simulink model "BCM_MBD_External_Lighting"  (R2020b)
settings: Solver=VariableStepAuto  StartTime=0.0  StopTime=50  RelTol=1e-3
undefined symbols (not defined in the file): sigbuilder_block
settings Model: Creator=99003151  LastModifiedBy=99003151

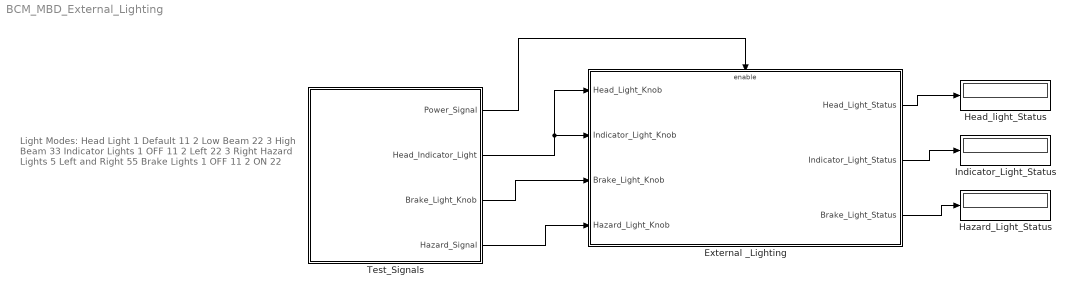
== system BCM_MBD_External_Lighting ==
  note: Light Modes:
      |
      | Head Light
      | 1
      | Default
      | 11
      |
      | 2
      | Low Beam
      | 22
      |
      | 3
      | High Beam
      | 33
      |
      | Indicator Lights
      | 1
      | OFF
      | 11
      |
      | 2
      | Left
      | 22
      |
      | 3
      | Right
      |
      | Hazard Lights
      | 5
      | Left and Right
      | 55
      |
      | Brake Lights
      | 1
      | OFF
      | 11
      |
      | 2
      | ON
      | 22
  External _Lighting : Subsystem  TreatAsAtomicUnit=on
  Hazard_Light_Status : Display
  Head_light_Status : Display
  Indicator_Light_Status : Display
  Test_Signals : Subsystem  Tag=STV Subsys  LoadFcn=sigbuilder_block('load');  StartFcn=sigbuilder_block('start');  StopFcn=sigbuilder_block('stop');  ClipboardFcn=sigbuilder_block('clipboard');  mask(Sigbuilder block){tuvar=[0:10]}
      mask help: Simulink:masks:SigbuilderBlock_MD
      mask init:
      | if ~strcmp(get_param(bdroot(gcbh),'SimulationStatus'),'stopped') tuvar = sigbuilder_block('maskInit'); end
      settings: CopyFcn=sigbuilder_block('copy');  DeleteFcn=sigbuilder_block('delete');  ModelCloseFcn=sigbuilder_block('modelClose');  PreSaveFcn=sigbuilder_block('preSave');  PauseFcn=sigbuilder_block('pause');  ContinueFcn=sigbuilder_block('continue');  NameChangeFcn=sigbuilder_block('namechange');  OpenFcn=sigbuilder_block('open',[437.6 153 550.4 359.25 ]);  CloseFcn=sigbuilder_block('close');
      mask Display: plot(0, 0, 100, 100,[2, 2, 32, 32, 2], [68, 8, 8, 68, 68],[32, 2], [38, 38], [32, 19, 2],[53, 60, 44], [32, 17, 17, 2],[16, 16, 31, 31]);txt = getActiveGroup(gcbh);text(2, 100, txt,'verticalAlignment', 'top');
  wires:
  External _Lighting/1(Head_Light_Status) -> Head_light_Status/1
  External _Lighting/2(Indicator_Light_Status) -> Indicator_Light_Status/1
  External _Lighting/3(Brake_Light_Status) -> Hazard_Light_Status/1
  Test_Signals/2(Head_Indicator_Light) -> External _Lighting/2(Indicator_Light_Knob), External _Lighting/1(Head_Light_Knob)
  Test_Signals/3(Brake_Light_Knob) -> External _Lighting/3(Brake_Light_Knob)
  Test_Signals/1(Power_Signal) -> External _Lighting/Enable
  Test_Signals/4(Hazard_Signal) -> External _Lighting/4(Hazard_Light_Knob)

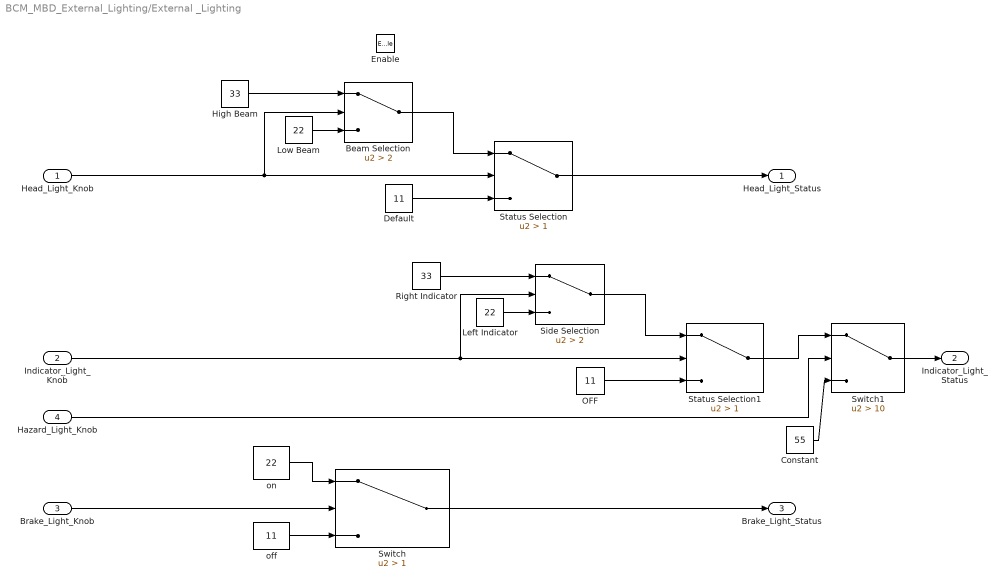
== system BCM_MBD_External_Lighting/External _Lighting ==
  Head_Light_Knob : Inport
  Indicator_Light_Knob : Inport  Port=2
  Brake_Light_Knob : Inport  Port=3
  Hazard_Light_Knob : Inport  Port=4
  Enable : EnablePort
  Beam Selection : Switch  Criteria=u2 > Threshold  Threshold=2
  Constant : Constant  Value=55
  Default : Constant  Value=11
  High Beam : Constant  Value=33
  Left Indicator : Constant  Value=22
  Low Beam : Constant  Value=22
  OFF : Constant  Value=11
  Right Indicator : Constant  Value=33
  Side Selection : Switch  Criteria=u2 > Threshold  Threshold=2
  Status Selection : Switch  Criteria=u2 > Threshold  Threshold=1
  Status Selection1 : Switch  Criteria=u2 > Threshold  Threshold=1
  Switch : Switch  Criteria=u2 > Threshold  Threshold=1
  Switch1 : Switch  Criteria=u2 > Threshold  Threshold=10
  off : Constant  Value=11
  on : Constant  Value=22
  Head_Light_Status : Outport
  Indicator_Light_Status : Outport  Port=2
  Brake_Light_Status : Outport  Port=3
  wires:
  Head_Light_Knob/1 -> Beam Selection/2, Status Selection/2
  Status Selection/1 -> Head_Light_Status/1
  Default/1 -> Status Selection/3
  High Beam/1 -> Beam Selection/1
  Low Beam/1 -> Beam Selection/3
  Beam Selection/1 -> Status Selection/1
  Right Indicator/1 -> Side Selection/1
  Side Selection/1 -> Status Selection1/1
  Left Indicator/1 -> Side Selection/3
  OFF/1 -> Status Selection1/3
  Brake_Light_Knob/1 -> Switch/2
  on/1 -> Switch/1
  off/1 -> Switch/3
  Switch/1 -> Brake_Light_Status/1
  Hazard_Light_Knob/1 -> Switch1/2
  Constant/1 -> Switch1/3
  Indicator_Light_Knob/1 -> Side Selection/2, Status Selection1/2
  Switch1/1 -> Indicator_Light_Status/1
  Status Selection1/1 -> Switch1/1

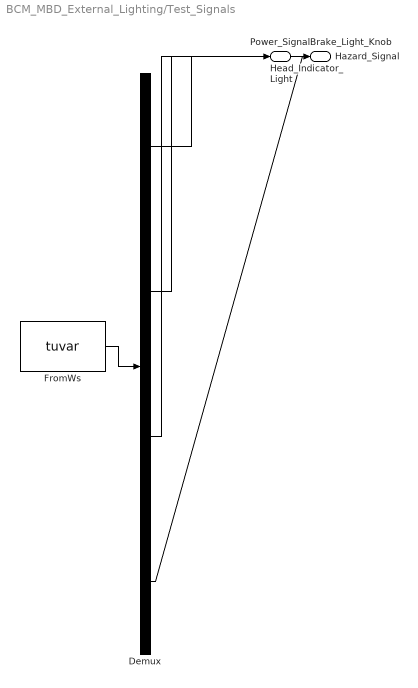
== system BCM_MBD_External_Lighting/Test_Signals ==
  Demux : Demux  Tag=STV Demux
      settings: DisplayOption=none
  FromWs : FromWorkspace  Tag=STV FromWs  VariableName=tuvar
      SigBuilderData=|
      | common.afterFinalStr = 'Extrapolate'
      | common.sampleTime = 0
      | dataSet.timeRange = [0 10]
      | dataSet.name = 'Group 1'
      | sbobj.Groups.Name = 'Group 1'
      | sbobj.Groups.Signals(1).Name = 'Power_Signal'
      | sbobj.Groups.Signals(1).XData = [0 3 3 10]
      | sbobj.Groups.Signals(1).YData = [0 0 1 1]
      | sbobj.Groups.Signals(2).Name = 'Head_Indicator_Light'
      | sbobj.Groups.Signals(2).XData = [0 1 1 2 2 3 3 3.99 4 4.99 5 5.98 6 7 7 7.98 8 9 9 10]
      | sbobj.Groups.Signals(2).YData = [1 1 2 2 3 3 1 1 2 2 3 3 1 1 2 2 3 3 1 1]
      | sbobj.Groups.Signals(3).Name = 'Brake_Light_Knob'
      | sbobj.Groups.Signals(3).XData = [0 1 1 2 2 3 3 3.99 4 4.99 5 10]
      | sbobj.Groups.Signals(3).YData = [1 1 2 2 1 1 2 2 1 1 2 2]
      | sbobj.Groups.Signals(4).Name = 'Hazard_Signal'
      | sbobj.Groups.Signals(4).XData = [0 6 6 9 9 10]
      | sbobj.Groups.Signals(4).YData = [0 0 1 1 0 0]
  Power_Signal : Outport  Tag=STV Outport
  Head_Indicator_Light : Outport  Tag=STV Outport  Port=2
  Brake_Light_Knob : Outport  Tag=STV Outport  Port=3
  Hazard_Signal : Outport  Tag=STV Outport  Port=4
  wires:
  FromWs/1 -> Demux/1
  Demux/1 -> Power_Signal/1
  Demux/2 -> Head_Indicator_Light/1
  Demux/3 -> Brake_Light_Knob/1
  Demux/4 -> Hazard_Signal/1
